simulink model "serialtest2"  (R2014b)
settings: Solver=ode45  StartTime=0.0  StopTime=inf  RelTol=1e-3
undefined symbols (not defined in the file): CR, fdesignblkfcn, gcbh, rpy2tr, serial, T
libraries: roblocks x6, instrumentlib x2, dspinverses x1, dspmtrx3 x1, simulink x1, dspmathops x1
settings Model: BufferReuse=off  Creator=Edoardo  LastModifiedBy=Edoardo
settings OptimizationCC: BlockReduction=off  ConditionallyExecuteInputs=off  OptimizeBlockIOStorage=off  BufferReuse=off  GlobalBufferReuse=off  ExpressionFolding=off  LocalBlockOutputs=off

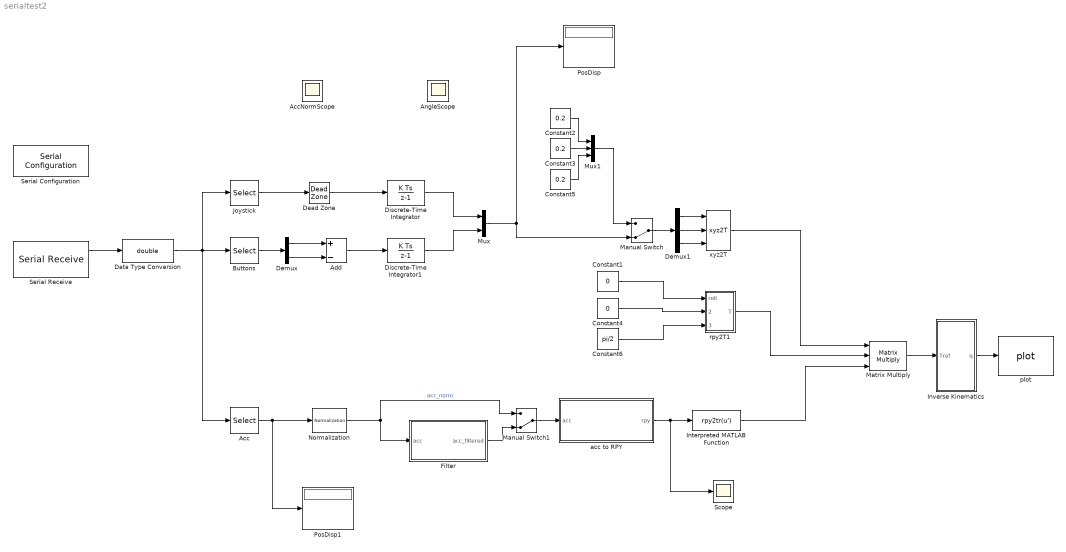
== system serialtest2 ==
  Acc : Selector  InputPortWidth=7  Indices=[5 6 7]
  AccNormScope : Scope
      settings: Floating=on  ShowLegends=on  YMin=0  YMax=1
  Add : Sum  Inputs=+-
  AngleScope : Scope
      settings: Floating=on  ShowLegends=on  YMin=-0.2  YMax=1.6
  Buttons : Selector  InputPortWidth=7  Indices=[3 4]
  Constant1 : Constant  Value=0
  Constant2 : Constant  Value=0.2
  Constant3 : Constant  Value=0.2
  Constant4 : Constant  Value=0
  Constant5 : Constant  Value=0.2
  Constant6 : Constant  Value=pi/2
  Data Type Conversion : DataTypeConversion  OutDataTypeStr=double
  Dead Zone : DeadZone  LowerValue=-20  UpperValue=20  SaturateOnIntegerOverflow=on
  Demux : Demux  Outputs=2
  Demux1 : Demux  Outputs=3
  Discrete-Time Integrator : DiscreteIntegrator  gainval=0.0002  InitialCondition=[0.2 0.2]  InitialConditionSetting=State (most efficient)  SampleTime=-1  LimitOutput=on  UpperSaturationLimit=0.5  LowerSaturationLimit=-0.5
  Discrete-Time Integrator1 : DiscreteIntegrator  gainval=0.02  InitialCondition=0.2  InitialConditionSetting=State (most efficient)  SampleTime=-1  LimitOutput=on  UpperSaturationLimit=0.6  LowerSaturationLimit=-0.6
  Filter : Subsystem
  Interpreted MATLAB Function : MATLABFcn  MATLABFcn=rpy2tr(u')  OutputDimensions=[4 4]  OutputSignalType=real  Output1D=off
  Inverse Kinematics : Subsystem  mask{Jd=0.02, K=5}
      mask prompts: Jd "Jacobian damping"; K "Error gain"
  Joystick : Selector  InputPortWidth=7  Indices=[1 2]
  Manual Switch : ManualSwitch  CurrentSetting=0
  Manual Switch1 : ManualSwitch  CurrentSetting=0
  Matrix Multiply : Product  Inputs=3  Multiplication=Matrix(*)
  Mux : Mux  Inputs=2
  Mux1 : Mux  Inputs=3
  Normalization : dspmathops/Normalization  NormType=2-norm  Bias=1e-10  NormOver=Each column  ColComp=on  Dimension=1  outputDataTypeStr=Inherit: Same as product output  outputLastDataTypeStr=Inherit: Same as product output  outputMin=[]  outputMax=[]  accumDataTypeStr=Inherit: Same as product output  accumLastDataTypeStr=Inherit: Same as product output  roundingMode=Floor  overflowMode=off
  PosDisp : Display
  PosDisp1 : Display
  Scope : Scope
      settings: SaveName=ScopeData2
  Serial Configuration : instrumentlib/Serial Configuration  Priority=-200000  ComPortMenu=COM5  ComPort=COM5  ObjConstructor=serial('COM5');  BaudRate=115200  DataBits=8  Parity=none  StopBits=1  FlowControl=none  Timeout=10  ByteOrder=LittleEndian
  Serial Receive : instrumentlib/Serial Receive  ComPortMenu=COM5  ComPort=COM5  ObjConstructor=serial('COM5');  Header=\a  Terminator=CR ('\r')  DataSize=7  DataType=int16  EnableBlockingMode=off  ActionDataUnavailable=Output last received value  CustomValue=0  SampleTime=0.1
  acc to RPY : Subsystem
  plot : roblocks/Robot Graphics/plot  robot=p560  fps=25  holdplot=on
  rpy2T1 : Subsystem  AncestorBlock=roblocks/Transform Conversion/rpy2T
      mask help: Convert roll/pitch/yaw angles to transform.
      mask Help:
      | Convert roll/pitch/yaw angles to homogeneous transformation.
      | 
      | 
      | <b>Inputs::</b>
      | 
      | roll (1x1) roll angle [rad]
      | pitch (1x1) pitch angle [rad]
      | yaw (1x1) yaw angle [rad]
      | 
      | 
      | <b>Outputs::</b>
      | 
      | T (4x4) the attitude as a homogeneous transformation
      | 
      | <b>Notes::</b>
      | 
      | - Axis rotation order is x-y-z (aerospace convention).
      | - Wrapper for the Toolbox function rpy2tr().
  xyz2T : roblocks/Transform Conversion/xyz2T
  wires:
  Serial Receive/1 -> Data Type Conversion/1
  Joystick/1 -> Dead Zone/1
  Dead Zone/1 -> Discrete-Time Integrator/1
  Data Type Conversion/1 -> Joystick/1, Acc/1, Buttons/1
  Buttons/1 -> Demux/1
  Demux/1 -> Add/1
  Demux/2 -> Add/2
  Add/1 -> Discrete-Time Integrator1/1
  Mux/1 -> Manual Switch/2, PosDisp/1
  Discrete-Time Integrator/1 -> Mux/1
  Discrete-Time Integrator1/1 -> Mux/2
  Acc/1 -> PosDisp1/1, Normalization/1
  Inverse Kinematics/1(q) -> plot/1
  xyz2T/1 -> Matrix Multiply/1
  Matrix Multiply/1 -> Inverse Kinematics/1(Tref)
  Normalization/1 -> Manual Switch1/1, Filter/1(acc)  "acc_norm"
  acc to RPY/1(rpy) -> Scope/1, Interpreted MATLAB Function/1
  Demux1/3 -> xyz2T/3
  Demux1/2 -> xyz2T/2
  Demux1/1 -> xyz2T/1
  Constant5/1 -> Mux1/3
  Constant3/1 -> Mux1/2
  Constant2/1 -> Mux1/1
  Manual Switch/1 -> Demux1/1
  Filter/1(acc_filtered) -> Manual Switch1/2
  Manual Switch1/1 -> acc to RPY/1(acc)
  Mux1/1 -> Manual Switch/1
  Interpreted MATLAB Function/1 -> Matrix Multiply/3
  rpy2T1/1(T) -> Matrix Multiply/2
  Constant6/1 -> rpy2T1/3(yaw)
  Constant4/1 -> rpy2T1/2(pitch)
  Constant1/1 -> rpy2T1/1(roll)

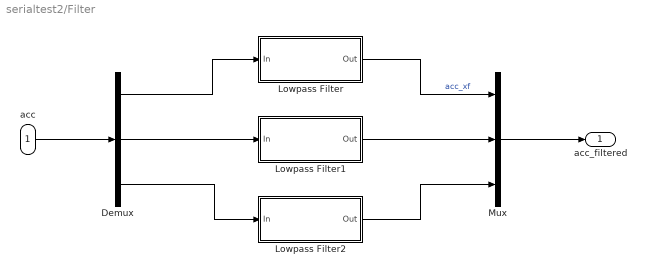
== system serialtest2/Filter ==
  acc : Inport
  Demux : Demux  Outputs=3
  Lowpass Filter : Subsystem  DialogController=fdesignblkfcn  InitFcn=fdesignblkfcn(gcbh, {'InitFcn'});  mask(Lowpass Filter){}
      mask help: Design a lowpass filter
      settings: CopyFcn=fdesignblkfcn(gcbh, {'CopyFcn'});
      mask Help: helpview(mapfilelocation('dsp'), 'dsplowpassfilter');
      mask Display: disp('Lowpass')
  Lowpass Filter1 : Subsystem  DialogController=fdesignblkfcn  InitFcn=fdesignblkfcn(gcbh, {'InitFcn'});  mask(Lowpass Filter){}
      mask help: Design a lowpass filter
      settings: CopyFcn=fdesignblkfcn(gcbh, {'CopyFcn'});
      mask Help: helpview(mapfilelocation('dsp'), 'dsplowpassfilter');
      mask Display: disp('Lowpass')
  Lowpass Filter2 : Subsystem  DialogController=fdesignblkfcn  InitFcn=fdesignblkfcn(gcbh, {'InitFcn'});  mask(Lowpass Filter){}
      mask help: Design a lowpass filter
      settings: CopyFcn=fdesignblkfcn(gcbh, {'CopyFcn'});
      mask Help: helpview(mapfilelocation('dsp'), 'dsplowpassfilter');
      mask Display: disp('Lowpass')
  Mux : Mux  Inputs=3
  acc_filtered : Outport
  wires:
  acc/1 -> Demux/1
  Demux/1 -> Lowpass Filter/1(In)
  Mux/1 -> acc_filtered/1
  Lowpass Filter/1(Out) -> Mux/1  "acc_xf"
  Demux/2 -> Lowpass Filter1/1(In)
  Demux/3 -> Lowpass Filter2/1(In)
  Lowpass Filter1/1(Out) -> Mux/2
  Lowpass Filter2/1(Out) -> Mux/3

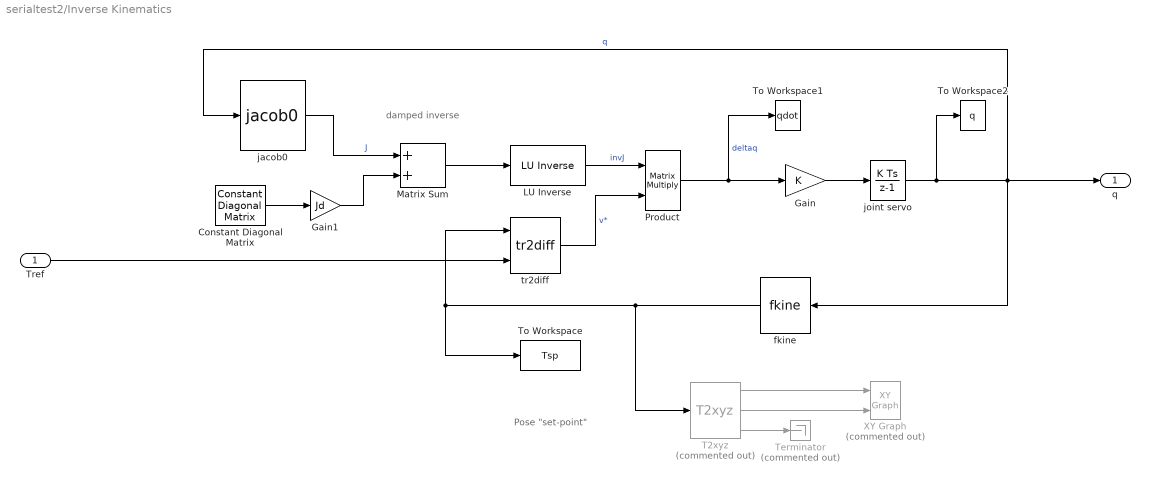
== system serialtest2/Inverse Kinematics ==
  note: Pose "set-point"
  note: damped inverse
  Tref : Inport
  " LU Inverse" : dspinverses/ LU Inverse
  Constant Diagonal Matrix : dspmtrx3/Constant Diagonal Matrix  q=ones(1,6)  frame=off  dataType=Inherit from 'Constant(s) along diagonal'  isSigned=on  wordLen=16  udDataType=sfix(16)  fracBitsMode=Best precision  numFracBits=15
  Gain : Gain  Gain=K  SaturateOnIntegerOverflow=on  OutDataTypeStr=Inherit: Same as input  ParamDataTypeStr=Inherit: Same as input
  Gain1 : Gain  Gain=Jd
  Matrix Sum : Sum
  Product : Product  Multiplication=Matrix(*)  SaturateOnIntegerOverflow=on  RndMeth=Zero  InputSameDT=on  OutDataTypeStr=Inherit: Same as first input
  T2xyz : roblocks/Transform Conversion/T2xyz  Commented=on
  Terminator : Terminator  Commented=on
  To Workspace : ToWorkspace  VariableName=Tsp  SampleTime=-1
  To Workspace1 : ToWorkspace  VariableName=qdot  SampleTime=-1
  To Workspace2 : ToWorkspace  VariableName=q  SampleTime=-1
  XY Graph : simulink/Sinks/XY Graph  Commented=on  xmin=-1  xmax=1  ymin=-1  ymax=1  st=-1
  fkine : roblocks/Kinematics/fkine  robot=robot
  "jacob0 " : roblocks/Kinematics/jacob0   robot=robot
  joint servo : DiscreteIntegrator  InitialCondition=qn'  SampleTime=T
  tr2diff : roblocks/Kinematics/tr2diff  robot=robot
  q : Outport
  wires:
  Constant Diagonal Matrix/1 -> Gain1/1
  Gain/1 -> joint servo/1
  " LU Inverse"/1 -> Product/1  "invJ"
  fkine/1 -> T2xyz/1, To Workspace/1, tr2diff/1
  Tref/1 -> tr2diff/2
  T2xyz/1 -> XY Graph/1
  Gain1/1 -> Matrix Sum/2
  "jacob0 "/1 -> Matrix Sum/1  "J"
  tr2diff/1 -> Product/2  "v*"
  T2xyz/2 -> XY Graph/2
  Matrix Sum/1 -> " LU Inverse"/1
  Product/1 -> To Workspace1/1, Gain/1  "deltaq"
  T2xyz/3 -> Terminator/1
  joint servo/1 -> To Workspace2/1, q/1, "jacob0 "/1, fkine/1  "q"

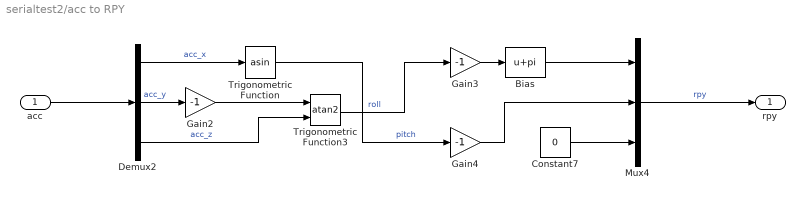
== system serialtest2/acc to RPY ==
  acc : Inport
  Bias : Bias  Bias=pi
  Constant7 : Constant  Value=0
  Demux2 : Demux  Outputs=3
  Gain2 : Gain  Gain=-1
  Gain3 : Gain  Gain=-1
  Gain4 : Gain  Gain=-1
  Mux4 : Mux  Inputs=3
  Trigonometric Function : Trigonometry  Operator=asin  OutputSignalType=real
  Trigonometric Function3 : Trigonometry  Operator=atan2  OutputSignalType=real
  rpy : Outport
  wires:
  Mux4/1 -> rpy/1  "rpy"
  Constant7/1 -> Mux4/3
  Gain4/1 -> Mux4/2
  Gain3/1 -> Bias/1
  Bias/1 -> Mux4/1
  Demux2/2 -> Gain2/1  "acc_y"
  Demux2/1 -> Trigonometric Function/1  "acc_x"
  Demux2/3 -> Trigonometric Function3/2  "acc_z"
  Gain2/1 -> Trigonometric Function3/1
  Trigonometric Function/1 -> Gain4/1  "pitch"
  acc/1 -> Demux2/1
  Trigonometric Function3/1 -> Gain3/1  "roll"

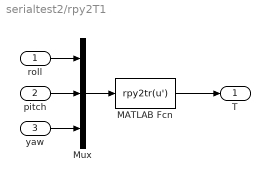
== system serialtest2/rpy2T1 ==
  roll : Inport
  pitch : Inport  Port=2
  yaw : Inport  Port=3
  MATLAB Fcn : MATLABFcn  MATLABFcn=rpy2tr(u')  OutputDimensions=[4 4]  Output1D=off
  Mux : Mux  Inputs=3
  T : Outport
  wires:
  yaw/1 -> Mux/3
  MATLAB Fcn/1 -> T/1
  Mux/1 -> MATLAB Fcn/1
  roll/1 -> Mux/1
  pitch/1 -> Mux/2

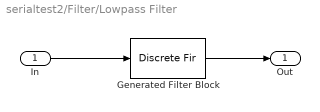
== system serialtest2/Filter/Lowpass Filter ==
  In : Inport
  Generated Filter Block : DiscreteFir  Tag=BlockMethodSubSystem  Coefficients=[0.012742901151903427 -0.056800702054434916 -0.059982833693567543 0.29300036476275532 0.57505703151959175 0.29300036476275532 -0.059982833693567543 -0.056800702054434916 0.012742901151903427]  InputProcessing=Columns as channels (frame based)
  Out : Outport
  wires:
  In/1 -> Generated Filter Block/1
  Generated Filter Block/1 -> Out/1

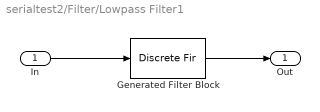
== system serialtest2/Filter/Lowpass Filter1 ==
  In : Inport
  Generated Filter Block : DiscreteFir  Tag=BlockMethodSubSystem  Coefficients=[0.012742901151903427 -0.056800702054434916 -0.059982833693567543 0.29300036476275532 0.57505703151959175 0.29300036476275532 -0.059982833693567543 -0.056800702054434916 0.012742901151903427]  InputProcessing=Columns as channels (frame based)
  Out : Outport
  wires:
  Generated Filter Block/1 -> Out/1
  In/1 -> Generated Filter Block/1

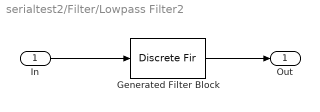
== system serialtest2/Filter/Lowpass Filter2 ==
  In : Inport
  Generated Filter Block : DiscreteFir  Tag=BlockMethodSubSystem  Coefficients=[0.012742901151903427 -0.056800702054434916 -0.059982833693567543 0.29300036476275532 0.57505703151959175 0.29300036476275532 -0.059982833693567543 -0.056800702054434916 0.012742901151903427]  InputProcessing=Columns as channels (frame based)
  Out : Outport
  wires:
  In/1 -> Generated Filter Block/1
  Generated Filter Block/1 -> Out/1
